simulink library "see_saw"  (R2013b)
settings: Solver=ode45  StartTime=0.0  StopTime=10.0  RelTol=1e-3
undefined symbols (not defined in the file): DiscIntNeverNeededParam, gcbh, K, R, realtime
libraries: legonxtlib x9
(part 1 of 2)
settings Model: Creator=mbiesiad  LastModifiedBy=grouleau

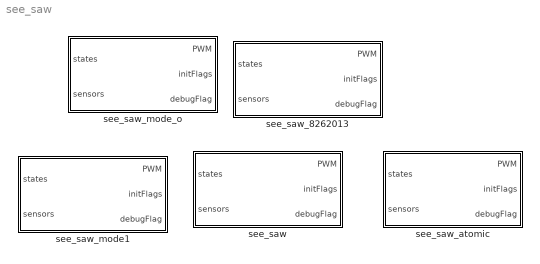
== system see_saw ==
  see_saw : Stateflow chart  TreatAsAtomicUnit=on
  see_saw_8262013 : Stateflow chart  TreatAsAtomicUnit=on
  see_saw_atomic : Stateflow chart  TreatAsAtomicUnit=on
  see_saw_mode1 : Stateflow chart  TreatAsAtomicUnit=on
  see_saw_mode_o : Stateflow chart  TreatAsAtomicUnit=on

== system see_saw/see_saw/see_saw_mode.DispTheta ==
  light : Inport  OutDataTypeStr=double  PortDimensions=1
  turningPWM : Inport  Port=2  OutDataTypeStr=double  PortDimensions=1
  f : TriggerPort  TriggerType=function-call
      settings: CopyFcn=Stateflow.SLINSF.SimulinkMan.removeBlockPreDeleteFcn  PreDeleteFcn=Stateflow.SLINSF.SimulinkMan.unsafePredeleteFcn
  Gain : Gain  Gain=100
  Gain1 : Gain  Gain=100
  LCD : legonxtlib/LCD  slcdStr=Theta  slcdLine=2  slcdFormat=Decimal
  LCD1 : Subsystem  InitFcn=realtime.validateBlock('LEGO MINDSTORMS NXT', gcbh, '')  mask(LEGO MINDSTORMS NXT LCD){slcdStr=turnPWM, slcdLine=3, slcdFormat=Decimal}
      mask prompts: slcdStr "Display label (maximum  8 characters):"; slcdLine "Display at line:"; slcdFormat "Display format:"
      mask help: Displays the numeric value from the block input port. The display truncates the input value to show only the integer portion. Use Display at line parameter to select the row. Use Display format parameter to select the format of the number: decimal or hexadecimal.
      mask init:
      | realtime.internal.nxtLcdSysCallback;
      mask Help: eval('realtime.helpView(''LEGO MINDSTORMS NXT'', ''legonxtlibnxtlcd'')')
      mask TypeOptions slcdLine: 1 | 2 | 3 | 4 | 5 | 6 | 7 | 8
      mask TypeOptions slcdFormat: Decimal | Hex
      mask Display:
      | [data, map]=imread('LCD.gif');pic=ind2rgb(data,map);image(pic,[0.32 0.25 0.35 0.55]);
      | lineText = sprintf('Line %d', slcdLine);
      | text(0.5, 0.15, lineText, 'horizontalAlignment', 'center');
      | port_label('input', 1, '');
      | color('blue');
      | text(0.65, 0.87, 'LEGO', 'horizontalAlignment', 'left');
  wires:
  Gain/1 -> LCD/1
  light/1 -> Gain/1
  Gain1/1 -> LCD1/1(In1)
  turningPWM/1 -> Gain1/1

== system see_saw/see_saw/see_saw_mode.Speak ==
  f : TriggerPort  TriggerType=function-call
      settings: CopyFcn=Stateflow.SLINSF.SimulinkMan.removeBlockPreDeleteFcn  PreDeleteFcn=Stateflow.SLINSF.SimulinkMan.unsafePredeleteFcn
  Constant : Constant  Value=50
  Speaker : legonxtlib/Speaker  sinputMode=Volume only  sspeakerFreq=800  sspeakerVolume=50  sspeakerDuration=100
  wires:
  Constant/1 -> Speaker/1

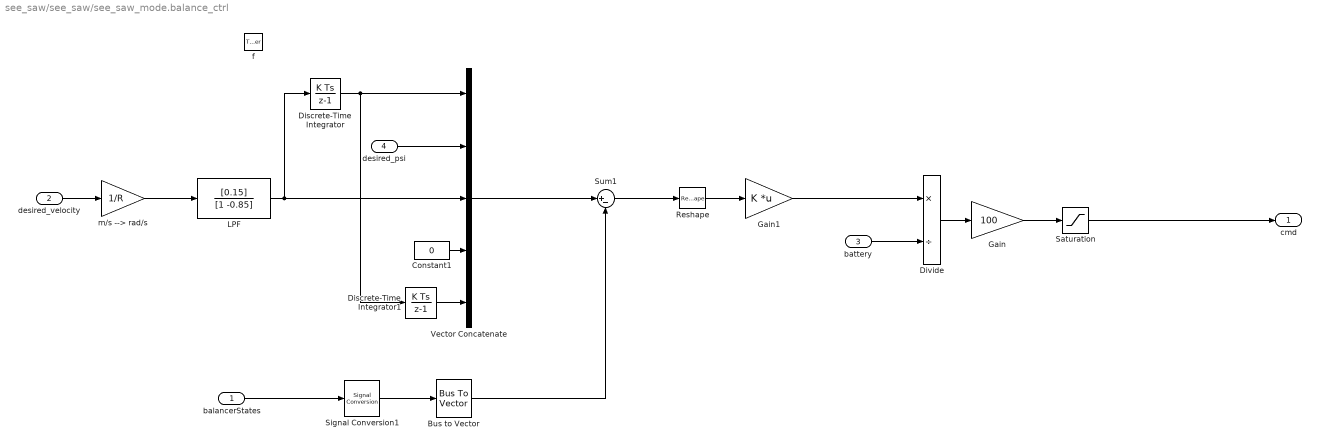
== system see_saw/see_saw/see_saw_mode.balance_ctrl ==
  balancerStates : Inport  OutDataTypeStr=Bus: Balancer_States_Bus  PortDimensions=1
  desired_velocity : Inport  Port=2  OutDataTypeStr=single  PortDimensions=1  BusOutputAsStruct=on
  battery : Inport  Port=3  OutDataTypeStr=double  PortDimensions=1
  desired_psi : Inport  Port=4  OutDataTypeStr=single  PortDimensions=1  BusOutputAsStruct=on
  f : TriggerPort  TriggerType=function-call
      settings: CopyFcn=Stateflow.SLINSF.SimulinkMan.removeBlockPreDeleteFcn  PreDeleteFcn=Stateflow.SLINSF.SimulinkMan.unsafePredeleteFcn
  Bus to Vector : BusToVector
  Constant1 : Constant  Value=0  OutDataTypeStr=single
  Discrete-Time Integrator : DiscreteIntegrator  SampleTime=-1  ICPrevOutput=DiscIntNeverNeededParam  ICPrevScaledInput=DiscIntNeverNeededParam
  Discrete-Time Integrator1 : DiscreteIntegrator  SampleTime=-1  ICPrevOutput=DiscIntNeverNeededParam  ICPrevScaledInput=DiscIntNeverNeededParam
  Divide : Product  Inputs=*/
  Gain : Gain  Gain=100
  Gain1 : Gain  Gain=K  Multiplication=Matrix(K*u)
  LPF : DiscreteFilter  Numerator=[0.15]  Denominator=[1 -0.85]
  Reshape : Reshape  OutputDimensionality=Column vector (2-D)
  Saturation : Saturate  UpperLimit=100  LowerLimit=-100  OutDataTypeStr=single
  Signal Conversion1 : SignalConversion  ConversionOutput=Virtual bus
  Sum1 : Sum  Inputs=|+-
  Vector Concatenate : Concatenate  NumInputs=5
  m/s --> rad/s : Gain  Gain=1/R
  cmd : Outport  OutDataTypeStr=single  PortDimensions=1  InitialOutput=0
  wires:
  Reshape/1 -> Gain1/1
  Sum1/1 -> Reshape/1
  desired_velocity/1 -> m/s --> rad/s/1
  Bus to Vector/1 -> Sum1/2
  balancerStates/1 -> Signal Conversion1/1
  Vector Concatenate/1 -> Sum1/1
  battery/1 -> Divide/2
  Saturation/1 -> cmd/1
  Gain1/1 -> Divide/1
  Gain/1 -> Saturation/1
  Divide/1 -> Gain/1
  Signal Conversion1/1 -> Bus to Vector/1
  m/s --> rad/s/1 -> LPF/1
  desired_psi/1 -> Vector Concatenate/2
  LPF/1 -> Discrete-Time Integrator/1, Vector Concatenate/3
  Constant1/1 -> Vector Concatenate/4
  Discrete-Time Integrator/1 -> Discrete-Time Integrator1/1, Vector Concatenate/1
  Discrete-Time Integrator1/1 -> Vector Concatenate/5

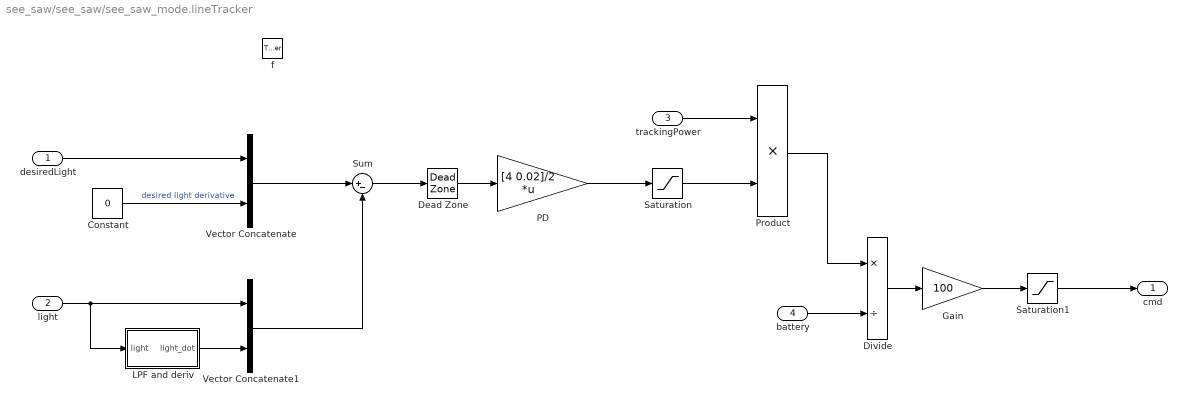
== system see_saw/see_saw/see_saw_mode.lineTracker ==
  desiredLight : Inport  OutDataTypeStr=single  PortDimensions=1
  light : Inport  Port=2  OutDataTypeStr=single  PortDimensions=1
  trackingPower : Inport  Port=3  OutDataTypeStr=single  PortDimensions=1
  battery : Inport  Port=4  OutDataTypeStr=double  PortDimensions=1
  f : TriggerPort  TriggerType=function-call
      settings: CopyFcn=Stateflow.SLINSF.SimulinkMan.removeBlockPreDeleteFcn  PreDeleteFcn=Stateflow.SLINSF.SimulinkMan.unsafePredeleteFcn
  Constant : Constant  Value=0  OutDataTypeStr=single
  Dead Zone : DeadZone  LowerValue=-0.02  UpperValue=0.02  SaturateOnIntegerOverflow=on
  Divide : Product  Inputs=*/
  Gain : Gain  Gain=100
  LPF and deriv : Subsystem
  PD : Gain  Gain="[4  0.02]/2"  Multiplication=Matrix(K*u)
  Product : Product
  Saturation : Saturate  UpperLimit=6  LowerLimit=-6
  Saturation1 : Saturate  UpperLimit=100  LowerLimit=-100  OutDataTypeStr=single
  Sum : Sum  Inputs=|+-
  Vector Concatenate : Concatenate
  Vector Concatenate1 : Concatenate
  cmd : Outport  OutDataTypeStr=single  PortDimensions=1
  wires:
  desiredLight/1 -> Vector Concatenate/1
  Constant/1 -> Vector Concatenate/2  "desired light derivative"
  LPF and deriv/1(light_dot) -> Vector Concatenate1/2
  light/1 -> LPF and deriv/1(light), Vector Concatenate1/1
  Vector Concatenate/1 -> Sum/1
  Vector Concatenate1/1 -> Sum/2
  Sum/1 -> Dead Zone/1
  Dead Zone/1 -> PD/1
  PD/1 -> Saturation/1
  Saturation/1 -> Product/2
  trackingPower/1 -> Product/1
  Product/1 -> Divide/1
  battery/1 -> Divide/2
  Gain/1 -> Saturation1/1
  Divide/1 -> Gain/1
  Saturation1/1 -> cmd/1

== system see_saw/see_saw/see_saw_mode.phiController ==
  phi : Inport  OutDataTypeStr=single  PortDimensions=1
  desiredPhi : Inport  Port=2  OutDataTypeStr=single  PortDimensions=1
  battery : Inport  Port=3  OutDataTypeStr=double  PortDimensions=1
  f : TriggerPort  TriggerType=function-call
      settings: CopyFcn=Stateflow.SLINSF.SimulinkMan.removeBlockPreDeleteFcn  PreDeleteFcn=Stateflow.SLINSF.SimulinkMan.unsafePredeleteFcn
  Divide : Product  Inputs=*/
  Gain : Gain  Gain=10
  Gain1 : Gain  Gain=100
  Saturation1 : Saturate  UpperLimit=100  LowerLimit=-100  OutDataTypeStr=single
  Sum : Sum  Inputs=|+-
  cmd : Outport
  wires:
  desiredPhi/1 -> Sum/1
  phi/1 -> Sum/2
  Sum/1 -> Gain/1
  battery/1 -> Divide/2
  Gain1/1 -> Saturation1/1
  Divide/1 -> Gain1/1
  Gain/1 -> Divide/1
  Saturation1/1 -> cmd/1

== system see_saw/see_saw/see_saw_mode.processLight ==
  rawLight : Inport  OutDataTypeStr=single  PortDimensions=1
  lightCalib : Inport  Port=2  OutDataTypeStr=Bus: Light_Bus  PortDimensions=1
  f : TriggerPort  TriggerType=function-call
      settings: CopyFcn=Stateflow.SLINSF.SimulinkMan.removeBlockPreDeleteFcn  PreDeleteFcn=Stateflow.SLINSF.SimulinkMan.unsafePredeleteFcn
  Bus Selector : BusSelector  OutputSignals=black,white
  Gain : Gain  Gain=0.3
  Gain1 : Gain  Gain=1/100
  Sum : Sum  Inputs=|+-
  Sum1 : Sum  Inputs=|++
  Sum2 : Sum  Inputs=|+-
  light : Outport
  wires:
  lightCalib/1 -> Bus Selector/1
  Bus Selector/1 -> Sum/1  "<black>"
  Bus Selector/2 -> Sum1/2, Sum/2  "<white>"
  Sum/1 -> Gain/1
  Gain/1 -> Sum1/1
  rawLight/1 -> Sum2/1
  Sum1/1 -> Sum2/2
  Sum2/1 -> Gain1/1
  Gain1/1 -> light/1

== system see_saw/see_saw/see_saw_mode.tail_controller ==
  note: Could be improved, PI for example
  current : Inport  OutDataTypeStr=single  PortDimensions=1
  desired : Inport  Port=2  OutDataTypeStr=single  PortDimensions=1
  f : TriggerPort  TriggerType=function-call
      settings: CopyFcn=Stateflow.SLINSF.SimulinkMan.removeBlockPreDeleteFcn  PreDeleteFcn=Stateflow.SLINSF.SimulinkMan.unsafePredeleteFcn
  Gain : Gain  Gain=250
  Saturation : Saturate  UpperLimit=100  LowerLimit=-100  OutDataTypeStr=single
  Sum : Sum  Inputs=|+-
  cmd : Outport  OutDataTypeStr=single  PortDimensions=1  InitialOutput=0
  wires:
  Sum/1 -> Gain/1
  current/1 -> Sum/2
  desired/1 -> Sum/1
  Gain/1 -> Saturation/1
  Saturation/1 -> cmd/1

== system see_saw/see_saw_8262013/see_saw_mode.DispTheta ==
  theta : Inport  OutDataTypeStr=double  PortDimensions=1
  f : TriggerPort  TriggerType=function-call
      settings: CopyFcn=Stateflow.SLINSF.SimulinkMan.removeBlockPreDeleteFcn  PreDeleteFcn=Stateflow.SLINSF.SimulinkMan.unsafePredeleteFcn
  Gain : Gain  Gain=100
  LCD : legonxtlib/LCD  slcdStr=Theta  slcdLine=2  slcdFormat=Decimal
  wires:
  theta/1 -> Gain/1
  Gain/1 -> LCD/1

== system see_saw/see_saw_8262013/see_saw_mode.Speak ==
  f : TriggerPort  TriggerType=function-call
      settings: CopyFcn=Stateflow.SLINSF.SimulinkMan.removeBlockPreDeleteFcn  PreDeleteFcn=Stateflow.SLINSF.SimulinkMan.unsafePredeleteFcn
  Constant : Constant  Value=50
  Speaker : legonxtlib/Speaker  sinputMode=Volume only  sspeakerFreq=800  sspeakerVolume=50  sspeakerDuration=100
  wires:
  Constant/1 -> Speaker/1

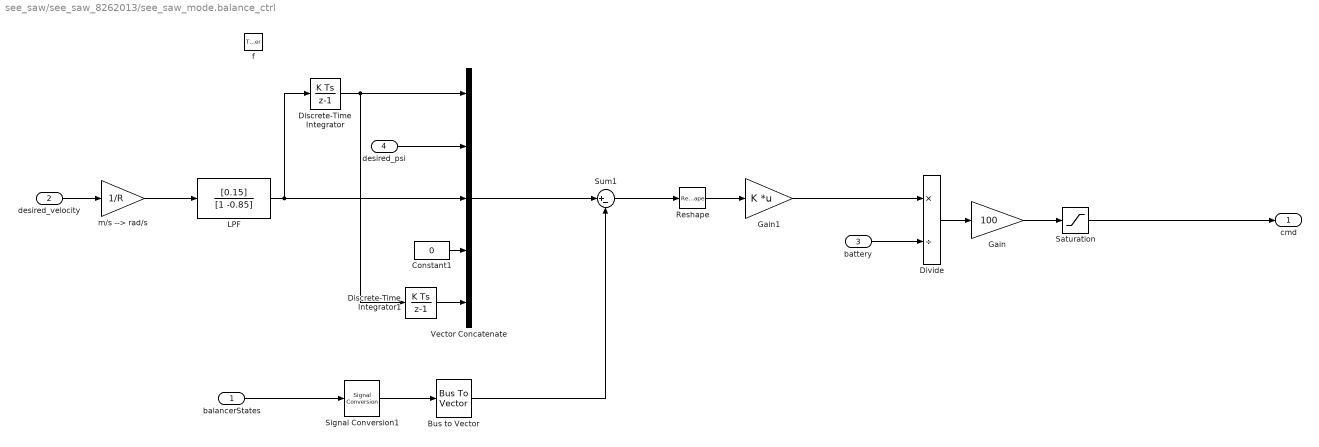
== system see_saw/see_saw_8262013/see_saw_mode.balance_ctrl ==
  balancerStates : Inport  OutDataTypeStr=Bus: Balancer_States_Bus  PortDimensions=1
  desired_velocity : Inport  Port=2  OutDataTypeStr=single  PortDimensions=1  BusOutputAsStruct=on
  battery : Inport  Port=3  OutDataTypeStr=double  PortDimensions=1
  desired_psi : Inport  Port=4  OutDataTypeStr=single  PortDimensions=1  BusOutputAsStruct=on
  f : TriggerPort  TriggerType=function-call
      settings: CopyFcn=Stateflow.SLINSF.SimulinkMan.removeBlockPreDeleteFcn  PreDeleteFcn=Stateflow.SLINSF.SimulinkMan.unsafePredeleteFcn
  Bus to Vector : BusToVector
  Constant1 : Constant  Value=0  OutDataTypeStr=single
  Discrete-Time Integrator : DiscreteIntegrator  SampleTime=-1  ICPrevOutput=DiscIntNeverNeededParam  ICPrevScaledInput=DiscIntNeverNeededParam
  Discrete-Time Integrator1 : DiscreteIntegrator  SampleTime=-1  ICPrevOutput=DiscIntNeverNeededParam  ICPrevScaledInput=DiscIntNeverNeededParam
  Divide : Product  Inputs=*/
  Gain : Gain  Gain=100
  Gain1 : Gain  Gain=K  Multiplication=Matrix(K*u)
  LPF : DiscreteFilter  Numerator=[0.15]  Denominator=[1 -0.85]
  Reshape : Reshape  OutputDimensionality=Column vector (2-D)
  Saturation : Saturate  UpperLimit=100  LowerLimit=-100  OutDataTypeStr=single
  Signal Conversion1 : SignalConversion  ConversionOutput=Virtual bus
  Sum1 : Sum  Inputs=|+-
  Vector Concatenate : Concatenate  NumInputs=5
  m/s --> rad/s : Gain  Gain=1/R
  cmd : Outport  OutDataTypeStr=single  PortDimensions=1  InitialOutput=0
  wires:
  Discrete-Time Integrator1/1 -> Vector Concatenate/5
  Discrete-Time Integrator/1 -> Vector Concatenate/1, Discrete-Time Integrator1/1
  Constant1/1 -> Vector Concatenate/4
  LPF/1 -> Vector Concatenate/3, Discrete-Time Integrator/1
  desired_psi/1 -> Vector Concatenate/2
  m/s --> rad/s/1 -> LPF/1
  Signal Conversion1/1 -> Bus to Vector/1
  Divide/1 -> Gain/1
  Gain/1 -> Saturation/1
  Gain1/1 -> Divide/1
  Saturation/1 -> cmd/1
  battery/1 -> Divide/2
  Vector Concatenate/1 -> Sum1/1
  balancerStates/1 -> Signal Conversion1/1
  Bus to Vector/1 -> Sum1/2
  desired_velocity/1 -> m/s --> rad/s/1
  Sum1/1 -> Reshape/1
  Reshape/1 -> Gain1/1

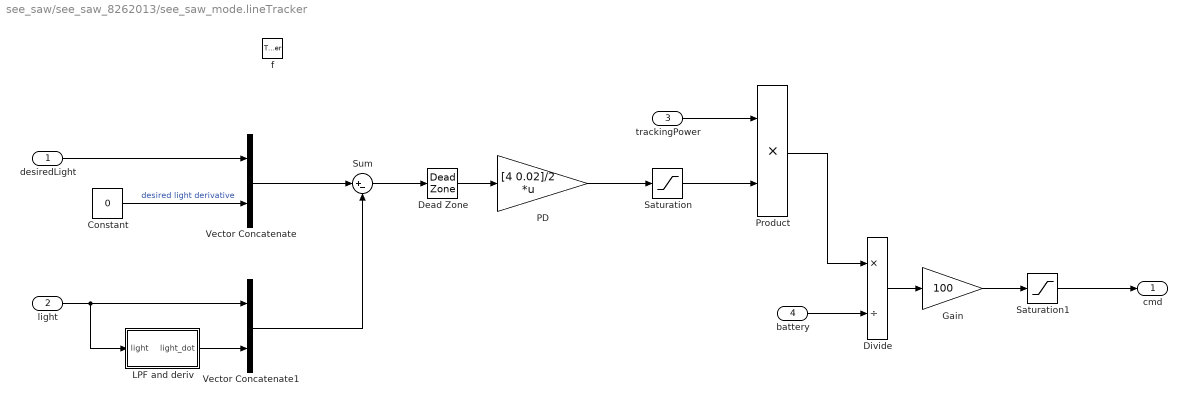
== system see_saw/see_saw_8262013/see_saw_mode.lineTracker ==
  desiredLight : Inport  OutDataTypeStr=single  PortDimensions=1
  light : Inport  Port=2  OutDataTypeStr=single  PortDimensions=1
  trackingPower : Inport  Port=3  OutDataTypeStr=single  PortDimensions=1
  battery : Inport  Port=4  OutDataTypeStr=double  PortDimensions=1
  f : TriggerPort  TriggerType=function-call
      settings: CopyFcn=Stateflow.SLINSF.SimulinkMan.removeBlockPreDeleteFcn  PreDeleteFcn=Stateflow.SLINSF.SimulinkMan.unsafePredeleteFcn
  Constant : Constant  Value=0  OutDataTypeStr=single
  Dead Zone : DeadZone  LowerValue=-0.02  UpperValue=0.02  SaturateOnIntegerOverflow=on
  Divide : Product  Inputs=*/
  Gain : Gain  Gain=100
  LPF and deriv : Subsystem
  PD : Gain  Gain="[4  0.02]/2"  Multiplication=Matrix(K*u)
  Product : Product
  Saturation : Saturate  UpperLimit=6  LowerLimit=-6
  Saturation1 : Saturate  UpperLimit=100  LowerLimit=-100  OutDataTypeStr=single
  Sum : Sum  Inputs=|+-
  Vector Concatenate : Concatenate
  Vector Concatenate1 : Concatenate
  cmd : Outport  OutDataTypeStr=single  PortDimensions=1
  wires:
  Saturation1/1 -> cmd/1
  Divide/1 -> Gain/1
  Gain/1 -> Saturation1/1
  battery/1 -> Divide/2
  Product/1 -> Divide/1
  trackingPower/1 -> Product/1
  Saturation/1 -> Product/2
  PD/1 -> Saturation/1
  Dead Zone/1 -> PD/1
  Sum/1 -> Dead Zone/1
  Vector Concatenate1/1 -> Sum/2
  Vector Concatenate/1 -> Sum/1
  light/1 -> Vector Concatenate1/1, LPF and deriv/1(light)
  LPF and deriv/1(light_dot) -> Vector Concatenate1/2
  Constant/1 -> Vector Concatenate/2  "desired light derivative"
  desiredLight/1 -> Vector Concatenate/1

== system see_saw/see_saw_8262013/see_saw_mode.phiController ==
  phi : Inport  OutDataTypeStr=single  PortDimensions=1
  desiredPhi : Inport  Port=2  OutDataTypeStr=single  PortDimensions=1
  battery : Inport  Port=3  OutDataTypeStr=double  PortDimensions=1
  f : TriggerPort  TriggerType=function-call
      settings: CopyFcn=Stateflow.SLINSF.SimulinkMan.removeBlockPreDeleteFcn  PreDeleteFcn=Stateflow.SLINSF.SimulinkMan.unsafePredeleteFcn
  Divide : Product  Inputs=*/
  Gain : Gain  Gain=10
  Gain1 : Gain  Gain=100
  Saturation1 : Saturate  UpperLimit=100  LowerLimit=-100  OutDataTypeStr=single
  Sum : Sum  Inputs=|+-
  cmd : Outport
  wires:
  Saturation1/1 -> cmd/1
  Gain/1 -> Divide/1
  Divide/1 -> Gain1/1
  Gain1/1 -> Saturation1/1
  battery/1 -> Divide/2
  Sum/1 -> Gain/1
  phi/1 -> Sum/2
  desiredPhi/1 -> Sum/1

== system see_saw/see_saw_8262013/see_saw_mode.processLight ==
  rawLight : Inport  OutDataTypeStr=single  PortDimensions=1
  lightCalib : Inport  Port=2  OutDataTypeStr=Bus: Light_Bus  PortDimensions=1
  f : TriggerPort  TriggerType=function-call
      settings: CopyFcn=Stateflow.SLINSF.SimulinkMan.removeBlockPreDeleteFcn  PreDeleteFcn=Stateflow.SLINSF.SimulinkMan.unsafePredeleteFcn
  Bus Selector : BusSelector  OutputSignals=black,white
  Gain : Gain  Gain=0.3
  Gain1 : Gain  Gain=1/100
  Sum : Sum  Inputs=|+-
  Sum1 : Sum  Inputs=|++
  Sum2 : Sum  Inputs=|+-
  light : Outport
  wires:
  Gain1/1 -> light/1
  Sum2/1 -> Gain1/1
  Sum1/1 -> Sum2/2
  rawLight/1 -> Sum2/1
  Gain/1 -> Sum1/1
  Sum/1 -> Gain/1
  Bus Selector/2 -> Sum/2, Sum1/2  "<white>"
  Bus Selector/1 -> Sum/1  "<black>"
  lightCalib/1 -> Bus Selector/1

== system see_saw/see_saw_8262013/see_saw_mode.tail_controller ==
  note: Could be improved, PI for example
  current : Inport  OutDataTypeStr=single  PortDimensions=1
  desired : Inport  Port=2  OutDataTypeStr=single  PortDimensions=1
  f : TriggerPort  TriggerType=function-call
      settings: CopyFcn=Stateflow.SLINSF.SimulinkMan.removeBlockPreDeleteFcn  PreDeleteFcn=Stateflow.SLINSF.SimulinkMan.unsafePredeleteFcn
  Gain : Gain  Gain=250
  Saturation : Saturate  UpperLimit=100  LowerLimit=-100  OutDataTypeStr=single
  Sum : Sum  Inputs=|+-
  cmd : Outport  OutDataTypeStr=single  PortDimensions=1  InitialOutput=0
  wires:
  Saturation/1 -> cmd/1
  Gain/1 -> Saturation/1
  desired/1 -> Sum/1
  current/1 -> Sum/2
  Sum/1 -> Gain/1

== system see_saw/see_saw_atomic/see_saw_mode.DispTheta ==
  light : Inport  OutDataTypeStr=double  PortDimensions=1
  turningPWM : Inport  Port=2  OutDataTypeStr=double  PortDimensions=1
  f : TriggerPort  TriggerType=function-call
      settings: CopyFcn=Stateflow.SLINSF.SimulinkMan.removeBlockPreDeleteFcn  PreDeleteFcn=Stateflow.SLINSF.SimulinkMan.unsafePredeleteFcn
  Gain : Gain  Gain=100
  Gain1 : Gain  Gain=100
  LCD : legonxtlib/LCD  slcdStr=Theta  slcdLine=2  slcdFormat=Decimal
  LCD1 : Subsystem  InitFcn=realtime.validateBlock('LEGO MINDSTORMS NXT', gcbh, '')  mask(LEGO MINDSTORMS NXT LCD){slcdStr=turnPWM, slcdLine=3, slcdFormat=Decimal}
      mask prompts: slcdStr "Display label (maximum  8 characters):"; slcdLine "Display at line:"; slcdFormat "Display format:"
      mask help: Displays the numeric value from the block input port. The display truncates the input value to show only the integer portion. Use Display at line parameter to select the row. Use Display format parameter to select the format of the number: decimal or hexadecimal.
      mask init:
      | realtime.internal.nxtLcdSysCallback;
      mask Help: eval('realtime.helpView(''LEGO MINDSTORMS NXT'', ''legonxtlibnxtlcd'')')
      mask TypeOptions slcdLine: 1 | 2 | 3 | 4 | 5 | 6 | 7 | 8
      mask TypeOptions slcdFormat: Decimal | Hex
      mask Display:
      | [data, map]=imread('LCD.gif');pic=ind2rgb(data,map);image(pic,[0.32 0.25 0.35 0.55]);
      | lineText = sprintf('Line %d', slcdLine);
      | text(0.5, 0.15, lineText, 'horizontalAlignment', 'center');
      | port_label('input', 1, '');
      | color('blue');
      | text(0.65, 0.87, 'LEGO', 'horizontalAlignment', 'left');
  wires:
  Gain/1 -> LCD/1
  light/1 -> Gain/1
  Gain1/1 -> LCD1/1(In1)
  turningPWM/1 -> Gain1/1

== system see_saw/see_saw_atomic/see_saw_mode.Speak ==
  f : TriggerPort  TriggerType=function-call
      settings: CopyFcn=Stateflow.SLINSF.SimulinkMan.removeBlockPreDeleteFcn  PreDeleteFcn=Stateflow.SLINSF.SimulinkMan.unsafePredeleteFcn
  Constant : Constant  Value=50
  Speaker : legonxtlib/Speaker  sinputMode=Volume only  sspeakerFreq=800  sspeakerVolume=50  sspeakerDuration=100
  wires:
  Constant/1 -> Speaker/1

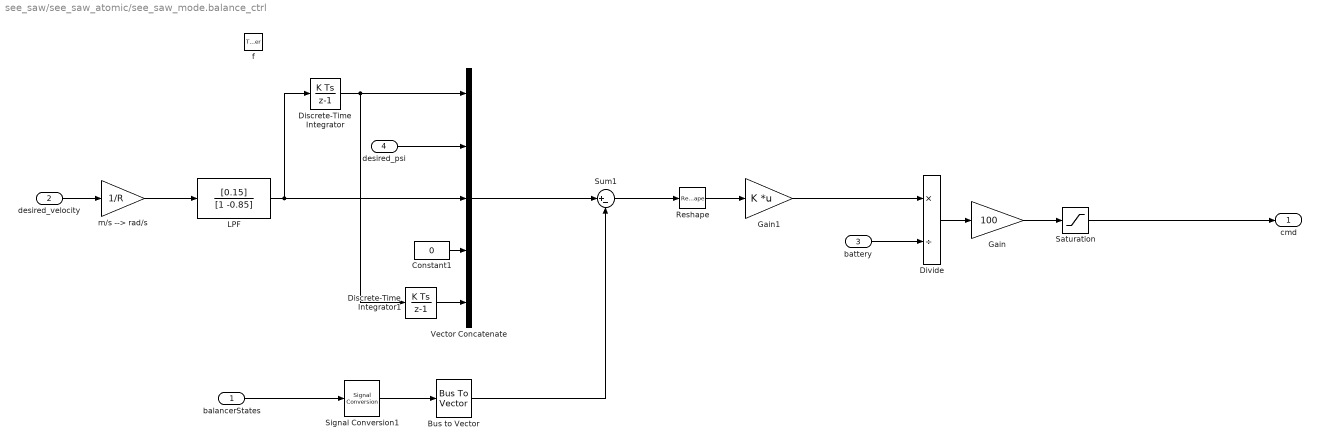
== system see_saw/see_saw_atomic/see_saw_mode.balance_ctrl ==
  balancerStates : Inport  OutDataTypeStr=Bus: Balancer_States_Bus  PortDimensions=1
  desired_velocity : Inport  Port=2  OutDataTypeStr=single  PortDimensions=1  BusOutputAsStruct=on
  battery : Inport  Port=3  OutDataTypeStr=double  PortDimensions=1
  desired_psi : Inport  Port=4  OutDataTypeStr=single  PortDimensions=1  BusOutputAsStruct=on
  f : TriggerPort  TriggerType=function-call
      settings: CopyFcn=Stateflow.SLINSF.SimulinkMan.removeBlockPreDeleteFcn  PreDeleteFcn=Stateflow.SLINSF.SimulinkMan.unsafePredeleteFcn
  Bus to Vector : BusToVector
  Constant1 : Constant  Value=0  OutDataTypeStr=single
  Discrete-Time Integrator : DiscreteIntegrator  SampleTime=-1  ICPrevOutput=DiscIntNeverNeededParam  ICPrevScaledInput=DiscIntNeverNeededParam
  Discrete-Time Integrator1 : DiscreteIntegrator  SampleTime=-1  ICPrevOutput=DiscIntNeverNeededParam  ICPrevScaledInput=DiscIntNeverNeededParam
  Divide : Product  Inputs=*/
  Gain : Gain  Gain=100
  Gain1 : Gain  Gain=K  Multiplication=Matrix(K*u)
  LPF : DiscreteFilter  Numerator=[0.15]  Denominator=[1 -0.85]
  Reshape : Reshape  OutputDimensionality=Column vector (2-D)
  Saturation : Saturate  UpperLimit=100  LowerLimit=-100  OutDataTypeStr=single
  Signal Conversion1 : SignalConversion  ConversionOutput=Virtual bus
  Sum1 : Sum  Inputs=|+-
  Vector Concatenate : Concatenate  NumInputs=5
  m/s --> rad/s : Gain  Gain=1/R
  cmd : Outport  OutDataTypeStr=single  PortDimensions=1  InitialOutput=0
  wires:
  Reshape/1 -> Gain1/1
  Sum1/1 -> Reshape/1
  desired_velocity/1 -> m/s --> rad/s/1
  Bus to Vector/1 -> Sum1/2
  balancerStates/1 -> Signal Conversion1/1
  Vector Concatenate/1 -> Sum1/1
  battery/1 -> Divide/2
  Saturation/1 -> cmd/1
  Gain1/1 -> Divide/1
  Gain/1 -> Saturation/1
  Divide/1 -> Gain/1
  Signal Conversion1/1 -> Bus to Vector/1
  m/s --> rad/s/1 -> LPF/1
  desired_psi/1 -> Vector Concatenate/2
  LPF/1 -> Discrete-Time Integrator/1, Vector Concatenate/3
  Constant1/1 -> Vector Concatenate/4
  Discrete-Time Integrator/1 -> Discrete-Time Integrator1/1, Vector Concatenate/1
  Discrete-Time Integrator1/1 -> Vector Concatenate/5

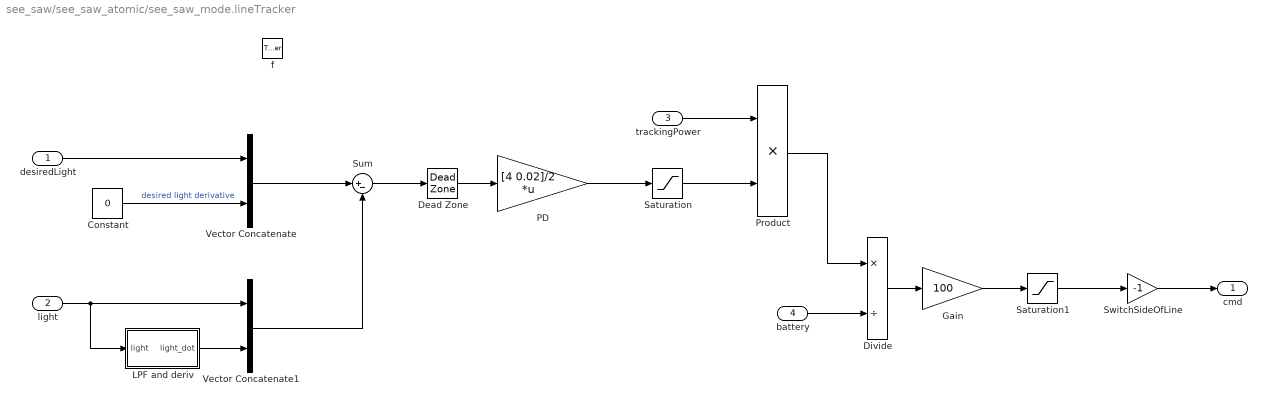
== system see_saw/see_saw_atomic/see_saw_mode.lineTracker ==
  desiredLight : Inport  OutDataTypeStr=single  PortDimensions=1
  light : Inport  Port=2  OutDataTypeStr=single  PortDimensions=1
  trackingPower : Inport  Port=3  OutDataTypeStr=single  PortDimensions=1
  battery : Inport  Port=4  OutDataTypeStr=double  PortDimensions=1
  f : TriggerPort  TriggerType=function-call
      settings: CopyFcn=Stateflow.SLINSF.SimulinkMan.removeBlockPreDeleteFcn  PreDeleteFcn=Stateflow.SLINSF.SimulinkMan.unsafePredeleteFcn
  Constant : Constant  Value=0  OutDataTypeStr=single
  Dead Zone : DeadZone  LowerValue=-0.02  UpperValue=0.02  SaturateOnIntegerOverflow=on
  Divide : Product  Inputs=*/
  Gain : Gain  Gain=100
  LPF and deriv : Subsystem
  PD : Gain  Gain="[4  0.02]/2"  Multiplication=Matrix(K*u)
  Product : Product
  Saturation : Saturate  UpperLimit=6  LowerLimit=-6
  Saturation1 : Saturate  UpperLimit=100  LowerLimit=-100  OutDataTypeStr=single
  Sum : Sum  Inputs=|+-
  SwitchSideOfLine : Gain  Gain=-1
  Vector Concatenate : Concatenate
  Vector Concatenate1 : Concatenate
  cmd : Outport  OutDataTypeStr=single  PortDimensions=1
  wires:
  SwitchSideOfLine/1 -> cmd/1
  desiredLight/1 -> Vector Concatenate/1
  Constant/1 -> Vector Concatenate/2  "desired light derivative"
  LPF and deriv/1(light_dot) -> Vector Concatenate1/2
  light/1 -> LPF and deriv/1(light), Vector Concatenate1/1
  Vector Concatenate/1 -> Sum/1
  Vector Concatenate1/1 -> Sum/2
  Sum/1 -> Dead Zone/1
  Dead Zone/1 -> PD/1
  PD/1 -> Saturation/1
  Saturation/1 -> Product/2
  trackingPower/1 -> Product/1
  Product/1 -> Divide/1
  battery/1 -> Divide/2
  Gain/1 -> Saturation1/1
  Divide/1 -> Gain/1
  Saturation1/1 -> SwitchSideOfLine/1

== system see_saw/see_saw_atomic/see_saw_mode.phiController ==
  phi : Inport  OutDataTypeStr=single  PortDimensions=1
  desiredPhi : Inport  Port=2  OutDataTypeStr=single  PortDimensions=1
  battery : Inport  Port=3  OutDataTypeStr=double  PortDimensions=1
  f : TriggerPort  TriggerType=function-call
      settings: CopyFcn=Stateflow.SLINSF.SimulinkMan.removeBlockPreDeleteFcn  PreDeleteFcn=Stateflow.SLINSF.SimulinkMan.unsafePredeleteFcn
  Divide : Product  Inputs=*/
  Gain : Gain  Gain=10
  Gain1 : Gain  Gain=100
  Saturation1 : Saturate  UpperLimit=100  LowerLimit=-100  OutDataTypeStr=single
  Sum : Sum  Inputs=|+-
  cmd : Outport
  wires:
  desiredPhi/1 -> Sum/1
  phi/1 -> Sum/2
  Sum/1 -> Gain/1
  battery/1 -> Divide/2
  Gain1/1 -> Saturation1/1
  Divide/1 -> Gain1/1
  Gain/1 -> Divide/1
  Saturation1/1 -> cmd/1

== system see_saw/see_saw_atomic/see_saw_mode.processLight ==
  rawLight : Inport  OutDataTypeStr=single  PortDimensions=1
  lightCalib : Inport  Port=2  OutDataTypeStr=Bus: Light_Bus  PortDimensions=1
  f : TriggerPort  TriggerType=function-call
      settings: CopyFcn=Stateflow.SLINSF.SimulinkMan.removeBlockPreDeleteFcn  PreDeleteFcn=Stateflow.SLINSF.SimulinkMan.unsafePredeleteFcn
  Bus Selector : BusSelector  OutputSignals=black,white
  Gain : Gain  Gain=0.3
  Gain1 : Gain  Gain=1/100
  Sum : Sum  Inputs=|+-
  Sum1 : Sum  Inputs=|++
  Sum2 : Sum  Inputs=|+-
  light : Outport
  wires:
  lightCalib/1 -> Bus Selector/1
  Bus Selector/1 -> Sum/1  "<black>"
  Bus Selector/2 -> Sum1/2, Sum/2  "<white>"
  Sum/1 -> Gain/1
  Gain/1 -> Sum1/1
  rawLight/1 -> Sum2/1
  Sum1/1 -> Sum2/2
  Sum2/1 -> Gain1/1
  Gain1/1 -> light/1

== system see_saw/see_saw_atomic/see_saw_mode.tail_controller ==
  note: Could be improved, PI for example
  current : Inport  OutDataTypeStr=single  PortDimensions=1
  desired : Inport  Port=2  OutDataTypeStr=single  PortDimensions=1
  f : TriggerPort  TriggerType=function-call
      settings: CopyFcn=Stateflow.SLINSF.SimulinkMan.removeBlockPreDeleteFcn  PreDeleteFcn=Stateflow.SLINSF.SimulinkMan.unsafePredeleteFcn
  Gain : Gain  Gain=250
  Saturation : Saturate  UpperLimit=100  LowerLimit=-100  OutDataTypeStr=single
  Sum : Sum  Inputs=|+-
  cmd : Outport  OutDataTypeStr=single  PortDimensions=1  InitialOutput=0
  wires:
  Sum/1 -> Gain/1
  current/1 -> Sum/2
  desired/1 -> Sum/1
  Gain/1 -> Saturation/1
  Saturation/1 -> cmd/1

== system see_saw/see_saw_mode1/see_saw_mode.Speak ==
  f : TriggerPort  TriggerType=function-call
      settings: CopyFcn=Stateflow.SLINSF.SimulinkMan.removeBlockPreDeleteFcn  PreDeleteFcn=Stateflow.SLINSF.SimulinkMan.unsafePredeleteFcn
  Constant : Constant  Value=50
  Speaker : legonxtlib/Speaker  sinputMode=Volume only  sspeakerFreq=800  sspeakerVolume=50  sspeakerDuration=100
  wires:
  Constant/1 -> Speaker/1

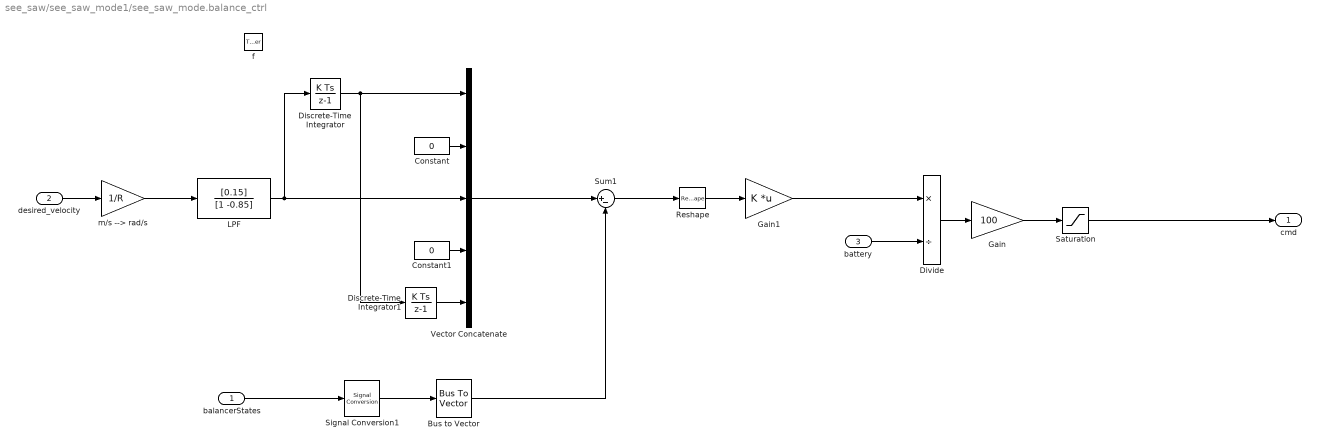
== system see_saw/see_saw_mode1/see_saw_mode.balance_ctrl ==
  balancerStates : Inport  OutDataTypeStr=Bus: Balancer_States_Bus  PortDimensions=1
  desired_velocity : Inport  Port=2  OutDataTypeStr=single  PortDimensions=1  BusOutputAsStruct=on
  battery : Inport  Port=3  OutDataTypeStr=double  PortDimensions=1
  f : TriggerPort  TriggerType=function-call
      settings: CopyFcn=Stateflow.SLINSF.SimulinkMan.removeBlockPreDeleteFcn  PreDeleteFcn=Stateflow.SLINSF.SimulinkMan.unsafePredeleteFcn
  Bus to Vector : BusToVector
  Constant : Constant  Value=0  OutDataTypeStr=single
  Constant1 : Constant  Value=0  OutDataTypeStr=single
  Discrete-Time Integrator : DiscreteIntegrator  SampleTime=-1  ICPrevOutput=DiscIntNeverNeededParam  ICPrevScaledInput=DiscIntNeverNeededParam
  Discrete-Time Integrator1 : DiscreteIntegrator  SampleTime=-1  ICPrevOutput=DiscIntNeverNeededParam  ICPrevScaledInput=DiscIntNeverNeededParam
  Divide : Product  Inputs=*/
  Gain : Gain  Gain=100
  Gain1 : Gain  Gain=K  Multiplication=Matrix(K*u)
  LPF : DiscreteFilter  Numerator=[0.15]  Denominator=[1 -0.85]
  Reshape : Reshape  OutputDimensionality=Column vector (2-D)
  Saturation : Saturate  UpperLimit=100  LowerLimit=-100  OutDataTypeStr=single
  Signal Conversion1 : SignalConversion  ConversionOutput=Virtual bus
  Sum1 : Sum  Inputs=|+-
  Vector Concatenate : Concatenate  NumInputs=5
  m/s --> rad/s : Gain  Gain=1/R
  cmd : Outport  OutDataTypeStr=single  PortDimensions=1  InitialOutput=0
  wires:
  Discrete-Time Integrator1/1 -> Vector Concatenate/5
  Discrete-Time Integrator/1 -> Vector Concatenate/1, Discrete-Time Integrator1/1
  Constant1/1 -> Vector Concatenate/4
  LPF/1 -> Vector Concatenate/3, Discrete-Time Integrator/1
  Constant/1 -> Vector Concatenate/2
  m/s --> rad/s/1 -> LPF/1
  Signal Conversion1/1 -> Bus to Vector/1
  Divide/1 -> Gain/1
  Gain/1 -> Saturation/1
  Gain1/1 -> Divide/1
  Saturation/1 -> cmd/1
  battery/1 -> Divide/2
  Vector Concatenate/1 -> Sum1/1
  balancerStates/1 -> Signal Conversion1/1
  Bus to Vector/1 -> Sum1/2
  desired_velocity/1 -> m/s --> rad/s/1
  Sum1/1 -> Reshape/1
  Reshape/1 -> Gain1/1

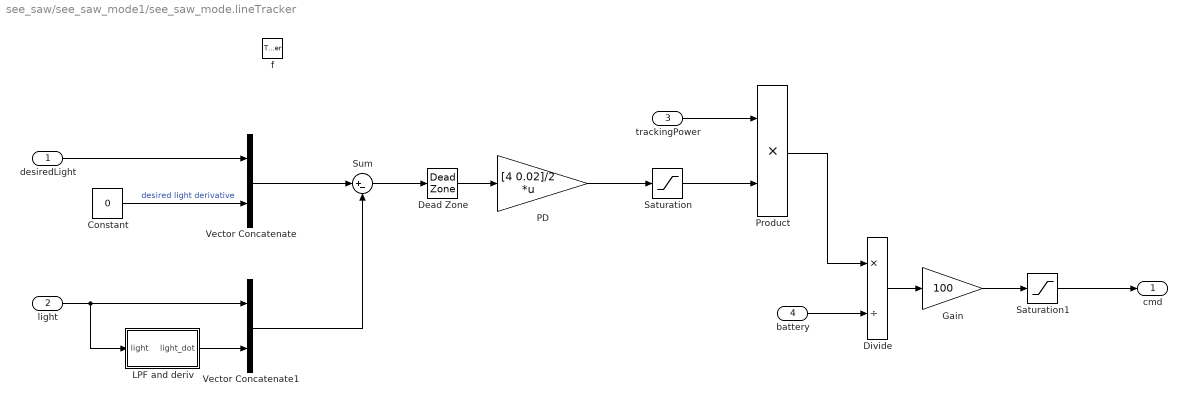
== system see_saw/see_saw_mode1/see_saw_mode.lineTracker ==
  desiredLight : Inport  OutDataTypeStr=single  PortDimensions=1
  light : Inport  Port=2  OutDataTypeStr=single  PortDimensions=1
  trackingPower : Inport  Port=3  OutDataTypeStr=single  PortDimensions=1
  battery : Inport  Port=4  OutDataTypeStr=double  PortDimensions=1
  f : TriggerPort  TriggerType=function-call
      settings: CopyFcn=Stateflow.SLINSF.SimulinkMan.removeBlockPreDeleteFcn  PreDeleteFcn=Stateflow.SLINSF.SimulinkMan.unsafePredeleteFcn
  Constant : Constant  Value=0  OutDataTypeStr=single
  Dead Zone : DeadZone  LowerValue=-0.02  UpperValue=0.02  SaturateOnIntegerOverflow=on
  Divide : Product  Inputs=*/
  Gain : Gain  Gain=100
  LPF and deriv : Subsystem
  PD : Gain  Gain="[4  0.02]/2"  Multiplication=Matrix(K*u)
  Product : Product
  Saturation : Saturate  UpperLimit=6  LowerLimit=-6
  Saturation1 : Saturate  UpperLimit=100  LowerLimit=-100  OutDataTypeStr=single
  Sum : Sum  Inputs=|+-
  Vector Concatenate : Concatenate
  Vector Concatenate1 : Concatenate
  cmd : Outport  OutDataTypeStr=single  PortDimensions=1
  wires:
  Saturation1/1 -> cmd/1
  Divide/1 -> Gain/1
  Gain/1 -> Saturation1/1
  battery/1 -> Divide/2
  Product/1 -> Divide/1
  trackingPower/1 -> Product/1
  Saturation/1 -> Product/2
  PD/1 -> Saturation/1
  Dead Zone/1 -> PD/1
  Sum/1 -> Dead Zone/1
  Vector Concatenate1/1 -> Sum/2
  Vector Concatenate/1 -> Sum/1
  light/1 -> Vector Concatenate1/1, LPF and deriv/1(light)
  LPF and deriv/1(light_dot) -> Vector Concatenate1/2
  Constant/1 -> Vector Concatenate/2  "desired light derivative"
  desiredLight/1 -> Vector Concatenate/1

== system see_saw/see_saw_mode1/see_saw_mode.phiController ==
  phi : Inport  OutDataTypeStr=single  PortDimensions=1
  desiredPhi : Inport  Port=2  OutDataTypeStr=single  PortDimensions=1
  battery : Inport  Port=3  OutDataTypeStr=double  PortDimensions=1
  f : TriggerPort  TriggerType=function-call
      settings: CopyFcn=Stateflow.SLINSF.SimulinkMan.removeBlockPreDeleteFcn  PreDeleteFcn=Stateflow.SLINSF.SimulinkMan.unsafePredeleteFcn
  Divide : Product  Inputs=*/
  Gain : Gain  Gain=10
  Gain1 : Gain  Gain=100
  Saturation1 : Saturate  UpperLimit=100  LowerLimit=-100  OutDataTypeStr=single
  Sum : Sum  Inputs=|+-
  cmd : Outport
  wires:
  Saturation1/1 -> cmd/1
  Gain/1 -> Divide/1
  Divide/1 -> Gain1/1
  Gain1/1 -> Saturation1/1
  battery/1 -> Divide/2
  Sum/1 -> Gain/1
  phi/1 -> Sum/2
  desiredPhi/1 -> Sum/1

== system see_saw/see_saw_mode1/see_saw_mode.processLight ==
  rawLight : Inport  OutDataTypeStr=single  PortDimensions=1
  lightCalib : Inport  Port=2  OutDataTypeStr=Bus: Light_Bus  PortDimensions=1
  f : TriggerPort  TriggerType=function-call
      settings: CopyFcn=Stateflow.SLINSF.SimulinkMan.removeBlockPreDeleteFcn  PreDeleteFcn=Stateflow.SLINSF.SimulinkMan.unsafePredeleteFcn
  Bus Selector : BusSelector  OutputSignals=black,white
  Gain : Gain  Gain=0.3
  Gain1 : Gain  Gain=1/100
  Sum : Sum  Inputs=|+-
  Sum1 : Sum  Inputs=|++
  Sum2 : Sum  Inputs=|+-
  light : Outport
  wires:
  Gain1/1 -> light/1
  Sum2/1 -> Gain1/1
  Sum1/1 -> Sum2/2
  rawLight/1 -> Sum2/1
  Gain/1 -> Sum1/1
  Sum/1 -> Gain/1
  Bus Selector/2 -> Sum/2, Sum1/2  "<white>"
  Bus Selector/1 -> Sum/1  "<black>"
  lightCalib/1 -> Bus Selector/1

== system see_saw/see_saw_mode1/see_saw_mode.tail_controller ==
  note: Could be improved, PI for example
  current : Inport  OutDataTypeStr=single  PortDimensions=1
  desired : Inport  Port=2  OutDataTypeStr=single  PortDimensions=1
  f : TriggerPort  TriggerType=function-call
      settings: CopyFcn=Stateflow.SLINSF.SimulinkMan.removeBlockPreDeleteFcn  PreDeleteFcn=Stateflow.SLINSF.SimulinkMan.unsafePredeleteFcn
  Gain : Gain  Gain=250
  Saturation : Saturate  UpperLimit=100  LowerLimit=-100  OutDataTypeStr=single
  Sum : Sum  Inputs=|+-
  cmd : Outport  OutDataTypeStr=single  PortDimensions=1  InitialOutput=0
  wires:
  Saturation/1 -> cmd/1
  Gain/1 -> Saturation/1
  desired/1 -> Sum/1
  current/1 -> Sum/2
  Sum/1 -> Gain/1

== system see_saw/see_saw_mode_o/see_saw_mode.DispTheta ==
  theta : Inport  OutDataTypeStr=double  PortDimensions=1
  f : TriggerPort  TriggerType=function-call
      settings: CopyFcn=Stateflow.SLINSF.SimulinkMan.removeBlockPreDeleteFcn  PreDeleteFcn=Stateflow.SLINSF.SimulinkMan.unsafePredeleteFcn
  Gain : Gain  Gain=100
  LCD : legonxtlib/LCD  slcdStr=Theta  slcdLine=2  slcdFormat=Decimal
  wires:
  Gain/1 -> LCD/1
  theta/1 -> Gain/1

== system see_saw/see_saw_mode_o/see_saw_mode.Speak ==
  f : TriggerPort  TriggerType=function-call
      settings: CopyFcn=Stateflow.SLINSF.SimulinkMan.removeBlockPreDeleteFcn  PreDeleteFcn=Stateflow.SLINSF.SimulinkMan.unsafePredeleteFcn
  Constant : Constant  Value=50
  Speaker : legonxtlib/Speaker  sinputMode=Volume only  sspeakerFreq=800  sspeakerVolume=50  sspeakerDuration=100
  wires:
  Constant/1 -> Speaker/1

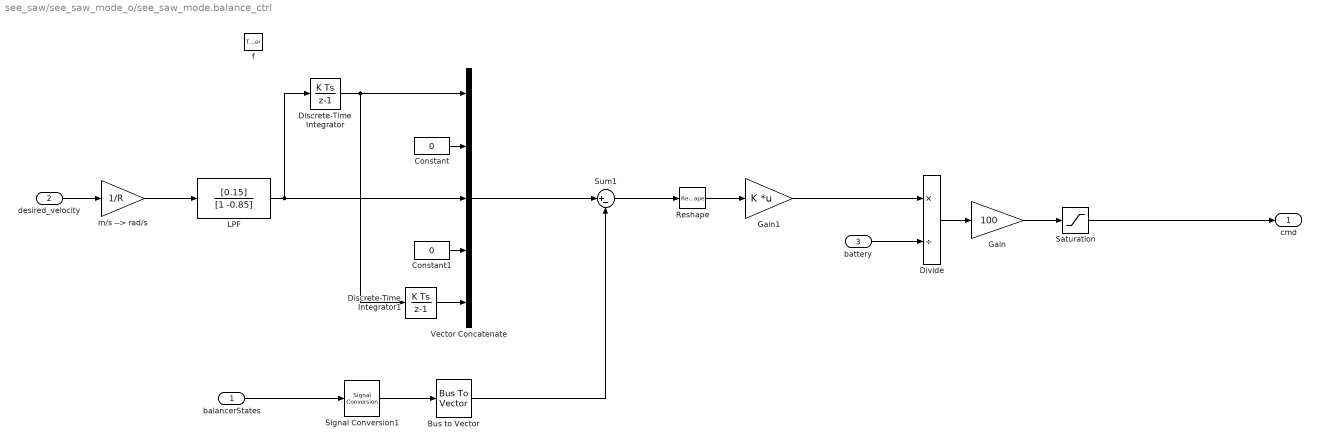
== system see_saw/see_saw_mode_o/see_saw_mode.balance_ctrl ==
  balancerStates : Inport  OutDataTypeStr=Bus: Balancer_States_Bus  PortDimensions=1
  desired_velocity : Inport  Port=2  OutDataTypeStr=single  PortDimensions=1  BusOutputAsStruct=on
  battery : Inport  Port=3  OutDataTypeStr=double  PortDimensions=1
  f : TriggerPort  TriggerType=function-call
      settings: CopyFcn=Stateflow.SLINSF.SimulinkMan.removeBlockPreDeleteFcn  PreDeleteFcn=Stateflow.SLINSF.SimulinkMan.unsafePredeleteFcn
  Bus to Vector : BusToVector
  Constant : Constant  Value=0  OutDataTypeStr=single
  Constant1 : Constant  Value=0  OutDataTypeStr=single
  Discrete-Time Integrator : DiscreteIntegrator  SampleTime=-1  ICPrevOutput=DiscIntNeverNeededParam  ICPrevScaledInput=DiscIntNeverNeededParam
  Discrete-Time Integrator1 : DiscreteIntegrator  SampleTime=-1  ICPrevOutput=DiscIntNeverNeededParam  ICPrevScaledInput=DiscIntNeverNeededParam
  Divide : Product  Inputs=*/
  Gain : Gain  Gain=100
  Gain1 : Gain  Gain=K  Multiplication=Matrix(K*u)
  LPF : DiscreteFilter  Numerator=[0.15]  Denominator=[1 -0.85]
  Reshape : Reshape  OutputDimensionality=Column vector (2-D)
  Saturation : Saturate  UpperLimit=100  LowerLimit=-100  OutDataTypeStr=single
  Signal Conversion1 : SignalConversion  ConversionOutput=Virtual bus
  Sum1 : Sum  Inputs=|+-
  Vector Concatenate : Concatenate  NumInputs=5
  m/s --> rad/s : Gain  Gain=1/R
  cmd : Outport  OutDataTypeStr=single  PortDimensions=1  InitialOutput=0
  wires:
  Reshape/1 -> Gain1/1
  Sum1/1 -> Reshape/1
  desired_velocity/1 -> m/s --> rad/s/1
  Bus to Vector/1 -> Sum1/2
  balancerStates/1 -> Signal Conversion1/1
  Vector Concatenate/1 -> Sum1/1
  battery/1 -> Divide/2
  Saturation/1 -> cmd/1
  Gain1/1 -> Divide/1
  Gain/1 -> Saturation/1
  Divide/1 -> Gain/1
  Signal Conversion1/1 -> Bus to Vector/1
  m/s --> rad/s/1 -> LPF/1
  Constant/1 -> Vector Concatenate/2
  LPF/1 -> Discrete-Time Integrator/1, Vector Concatenate/3
  Constant1/1 -> Vector Concatenate/4
  Discrete-Time Integrator/1 -> Discrete-Time Integrator1/1, Vector Concatenate/1
  Discrete-Time Integrator1/1 -> Vector Concatenate/5

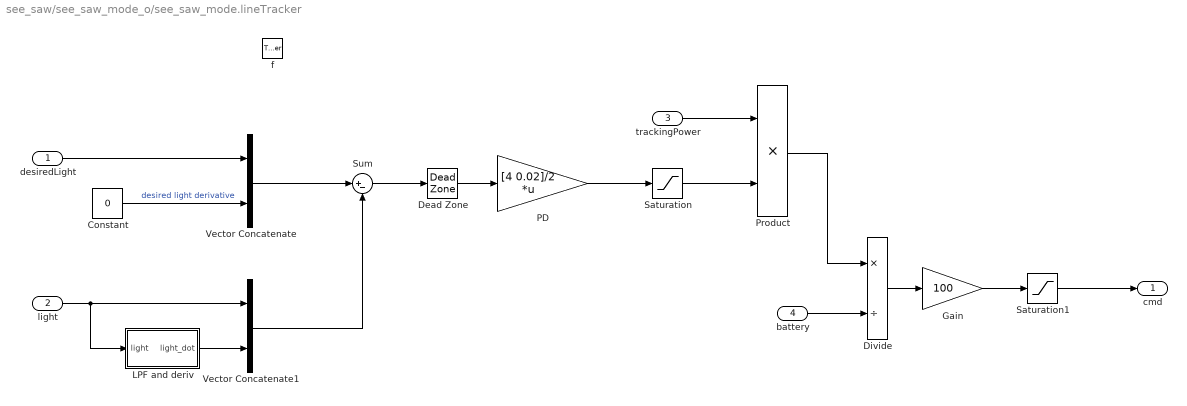
== system see_saw/see_saw_mode_o/see_saw_mode.lineTracker ==
  desiredLight : Inport  OutDataTypeStr=single  PortDimensions=1
  light : Inport  Port=2  OutDataTypeStr=single  PortDimensions=1
  trackingPower : Inport  Port=3  OutDataTypeStr=single  PortDimensions=1
  battery : Inport  Port=4  OutDataTypeStr=double  PortDimensions=1
  f : TriggerPort  TriggerType=function-call
      settings: CopyFcn=Stateflow.SLINSF.SimulinkMan.removeBlockPreDeleteFcn  PreDeleteFcn=Stateflow.SLINSF.SimulinkMan.unsafePredeleteFcn
  Constant : Constant  Value=0  OutDataTypeStr=single
  Dead Zone : DeadZone  LowerValue=-0.02  UpperValue=0.02  SaturateOnIntegerOverflow=on
  Divide : Product  Inputs=*/
  Gain : Gain  Gain=100
  LPF and deriv : Subsystem
  PD : Gain  Gain="[4  0.02]/2"  Multiplication=Matrix(K*u)
  Product : Product
  Saturation : Saturate  UpperLimit=6  LowerLimit=-6
  Saturation1 : Saturate  UpperLimit=100  LowerLimit=-100  OutDataTypeStr=single
  Sum : Sum  Inputs=|+-
  Vector Concatenate : Concatenate
  Vector Concatenate1 : Concatenate
  cmd : Outport  OutDataTypeStr=single  PortDimensions=1
  wires:
  desiredLight/1 -> Vector Concatenate/1
  Constant/1 -> Vector Concatenate/2  "desired light derivative"
  LPF and deriv/1(light_dot) -> Vector Concatenate1/2
  light/1 -> LPF and deriv/1(light), Vector Concatenate1/1
  Vector Concatenate/1 -> Sum/1
  Vector Concatenate1/1 -> Sum/2
  Sum/1 -> Dead Zone/1
  Dead Zone/1 -> PD/1
  PD/1 -> Saturation/1
  Saturation/1 -> Product/2
  trackingPower/1 -> Product/1
  Product/1 -> Divide/1
  battery/1 -> Divide/2
  Gain/1 -> Saturation1/1
  Divide/1 -> Gain/1
  Saturation1/1 -> cmd/1

== system see_saw/see_saw_mode_o/see_saw_mode.phiController ==
  phi : Inport  OutDataTypeStr=single  PortDimensions=1
  desiredPhi : Inport  Port=2  OutDataTypeStr=single  PortDimensions=1
  battery : Inport  Port=3  OutDataTypeStr=double  PortDimensions=1
  f : TriggerPort  TriggerType=function-call
      settings: CopyFcn=Stateflow.SLINSF.SimulinkMan.removeBlockPreDeleteFcn  PreDeleteFcn=Stateflow.SLINSF.SimulinkMan.unsafePredeleteFcn
  Divide : Product  Inputs=*/
  Gain : Gain  Gain=10
  Gain1 : Gain  Gain=100
  Saturation1 : Saturate  UpperLimit=100  LowerLimit=-100  OutDataTypeStr=single
  Sum : Sum  Inputs=|+-
  cmd : Outport
  wires:
  desiredPhi/1 -> Sum/1
  phi/1 -> Sum/2
  Sum/1 -> Gain/1
  battery/1 -> Divide/2
  Gain1/1 -> Saturation1/1
  Divide/1 -> Gain1/1
  Gain/1 -> Divide/1
  Saturation1/1 -> cmd/1

== system see_saw/see_saw_mode_o/see_saw_mode.processLight ==
  rawLight : Inport  OutDataTypeStr=single  PortDimensions=1
  lightCalib : Inport  Port=2  OutDataTypeStr=Bus: Light_Bus  PortDimensions=1
  f : TriggerPort  TriggerType=function-call
      settings: CopyFcn=Stateflow.SLINSF.SimulinkMan.removeBlockPreDeleteFcn  PreDeleteFcn=Stateflow.SLINSF.SimulinkMan.unsafePredeleteFcn
  Bus Selector : BusSelector  OutputSignals=black,white
  Gain : Gain  Gain=0.3
  Gain1 : Gain  Gain=1/100
  Sum : Sum  Inputs=|+-
  Sum1 : Sum  Inputs=|++
  Sum2 : Sum  Inputs=|+-
  light : Outport
  wires:
  lightCalib/1 -> Bus Selector/1
  Bus Selector/1 -> Sum/1  "<black>"
  Bus Selector/2 -> Sum1/2, Sum/2  "<white>"
  Sum/1 -> Gain/1
  Gain/1 -> Sum1/1
  rawLight/1 -> Sum2/1
  Sum1/1 -> Sum2/2
  Sum2/1 -> Gain1/1
  Gain1/1 -> light/1

== system see_saw/see_saw_mode_o/see_saw_mode.tail_controller ==
  note: Could be improved, PI for example
  current : Inport  OutDataTypeStr=single  PortDimensions=1
  desired : Inport  Port=2  OutDataTypeStr=single  PortDimensions=1
  f : TriggerPort  TriggerType=function-call
      settings: CopyFcn=Stateflow.SLINSF.SimulinkMan.removeBlockPreDeleteFcn  PreDeleteFcn=Stateflow.SLINSF.SimulinkMan.unsafePredeleteFcn
  Gain : Gain  Gain=250
  Saturation : Saturate  UpperLimit=100  LowerLimit=-100  OutDataTypeStr=single
  Sum : Sum  Inputs=|+-
  cmd : Outport  OutDataTypeStr=single  PortDimensions=1  InitialOutput=0
  wires:
  Sum/1 -> Gain/1
  current/1 -> Sum/2
  desired/1 -> Sum/1
  Gain/1 -> Saturation/1
  Saturation/1 -> cmd/1

== system see_saw/see_saw/see_saw_mode.DispTheta/LCD1 ==
  In1 : Inport
  Data Type Conversion : DataTypeConversion  OutDataTypeStr=int32
  LCD : S-Function  FunctionName=nxt_lcd  Parameters=lcdStr1, lcdLine, lcdFormat  EnableBusSupport=off  mask(NXT LCD){lcdStr=turnPWM, lcdLine=3, lcdFormat=Decimal}
      mask prompts: lcdStr "Prefix String (MAX 8 Characters):"; lcdLine "Display at Line:"; lcdFormat "Display Format:"
      mask help: Displays a number on NXT LCD screen
      mask init:
      | lcdStr1= [uint8(lcdStr) uint8(0)];
      mask TypeOptions lcdLine: 1 | 2 | 3 | 4 | 5 | 6 | 7 | 8
      mask TypeOptions lcdFormat: Decimal | Hex
      mask Display:
      | color('blue');
      | text(0.65, 0.87, 'LEGO', 'horizontalAlignment', 'left');
      | color('black');
      | port_label('input', 1, '');
  wires:
  Data Type Conversion/1 -> LCD/1
  In1/1 -> Data Type Conversion/1

== system see_saw/see_saw/see_saw_mode.lineTracker/LPF and deriv ==
  light : Inport
  Discrete Filter : DiscreteFilter  Numerator=[0.05]  Denominator=[1 -0.95]
  Gain : Gain  Gain=1/0.004
  Sum3 : Sum  Inputs=+-
  Unit Delay : UnitDelay  SampleTime=-1
  light_dot : Outport
  wires:
  light/1 -> Discrete Filter/1
  Discrete Filter/1 -> Gain/1
  Sum3/1 -> light_dot/1  "theta_dot_dot"
  Gain/1 -> Sum3/1, Unit Delay/1
  Unit Delay/1 -> Sum3/2

== system see_saw/see_saw_8262013/see_saw_mode.lineTracker/LPF and deriv ==
  light : Inport
  Discrete Filter : DiscreteFilter  Numerator=[0.05]  Denominator=[1 -0.95]
  Gain : Gain  Gain=1/0.004
  Sum3 : Sum  Inputs=+-
  Unit Delay : UnitDelay  SampleTime=-1
  light_dot : Outport
  wires:
  Unit Delay/1 -> Sum3/2
  Gain/1 -> Unit Delay/1, Sum3/1
  Sum3/1 -> light_dot/1  "theta_dot_dot"
  Discrete Filter/1 -> Gain/1
  light/1 -> Discrete Filter/1

== system see_saw/see_saw_atomic/see_saw_mode.DispTheta/LCD1 ==
  In1 : Inport
  Data Type Conversion : DataTypeConversion  OutDataTypeStr=int32
  LCD : S-Function  FunctionName=nxt_lcd  Parameters=lcdStr1, lcdLine, lcdFormat  EnableBusSupport=off  mask(NXT LCD){lcdStr=turnPWM, lcdLine=3, lcdFormat=Decimal}
      mask prompts: lcdStr "Prefix String (MAX 8 Characters):"; lcdLine "Display at Line:"; lcdFormat "Display Format:"
      mask help: Displays a number on NXT LCD screen
      mask init:
      | lcdStr1= [uint8(lcdStr) uint8(0)];
      mask TypeOptions lcdLine: 1 | 2 | 3 | 4 | 5 | 6 | 7 | 8
      mask TypeOptions lcdFormat: Decimal | Hex
      mask Display:
      | color('blue');
      | text(0.65, 0.87, 'LEGO', 'horizontalAlignment', 'left');
      | color('black');
      | port_label('input', 1, '');
  wires:
  Data Type Conversion/1 -> LCD/1
  In1/1 -> Data Type Conversion/1

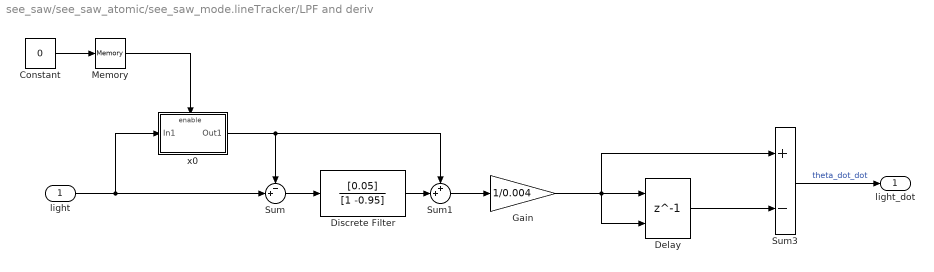
== system see_saw/see_saw_atomic/see_saw_mode.lineTracker/LPF and deriv ==
  light : Inport
  Constant : Constant  Value=0
  Delay : Delay  DelayLength=1  InitialConditionSource=Input port
      settings: InputPortMap=u0,p4
  Discrete Filter : DiscreteFilter  Numerator=[0.05]  Denominator=[1 -0.95]
  Gain : Gain  Gain=1/0.004
  Memory : Memory  X0=1  InheritSampleTime=on
  Sum : Sum  Inputs=-+|
  Sum1 : Sum  Inputs=++|
  Sum3 : Sum  Inputs=+-
  x0 : Subsystem  TreatAsAtomicUnit=on
  light_dot : Outport
  wires:
  Sum1/1 -> Gain/1
  Discrete Filter/1 -> Sum1/2
  x0/1(Out1) -> Sum/1, Sum1/1
  Sum/1 -> Discrete Filter/1
  Memory/1 -> x0/Enable
  Constant/1 -> Memory/1
  light/1 -> x0/1(In1), Sum/2
  Sum3/1 -> light_dot/1  "theta_dot_dot"
  Gain/1 -> Sum3/1, Delay/1, Delay/2
  Delay/1 -> Sum3/2

== system see_saw/see_saw_mode1/see_saw_mode.lineTracker/LPF and deriv ==
  light : Inport
  Discrete Filter : DiscreteFilter  Numerator=[0.05]  Denominator=[1 -0.95]
  Gain : Gain  Gain=1/0.004
  Sum3 : Sum  Inputs=+-
  Unit Delay : UnitDelay  SampleTime=-1
  light_dot : Outport
  wires:
  Unit Delay/1 -> Sum3/2
  Gain/1 -> Unit Delay/1, Sum3/1
  Sum3/1 -> light_dot/1  "theta_dot_dot"
  Discrete Filter/1 -> Gain/1
  light/1 -> Discrete Filter/1

== system see_saw/see_saw_mode_o/see_saw_mode.lineTracker/LPF and deriv ==
  light : Inport
  Discrete Filter : DiscreteFilter  Numerator=[0.05]  Denominator=[1 -0.95]
  Gain : Gain  Gain=1/0.004
  Sum3 : Sum  Inputs=+-
  Unit Delay : UnitDelay  SampleTime=-1
  light_dot : Outport
  wires:
  light/1 -> Discrete Filter/1
  Discrete Filter/1 -> Gain/1
  Sum3/1 -> light_dot/1  "theta_dot_dot"
  Gain/1 -> Sum3/1, Unit Delay/1
  Unit Delay/1 -> Sum3/2

== system see_saw/see_saw_atomic/see_saw_mode.lineTracker/LPF and deriv/x0 ==
  In1 : Inport
  Enable : EnablePort
  Out1 : Outport  InitialOutput=0
  wires:
  In1/1 -> Out1/1

== stateflow chart see_saw/see_saw_mode1 ==
  state see_saw_mode
    entry:
    desired_tail = single(1.6);
    during:
    normalizedLight = processLight(sensors.light,lightCalib);
    PWM.tail = tail_controller(sensors.theta_T, desired_tail);
    state light = processLight(rawLight,lightCalib) [function]
    state StandUp
      entry: debugFlag = uint16(602);
      initFlags.theta = single(1);
      initFlags.gyroReset = single(1);
      during:
      desired_tail = desired_tail + single(0.0008);
    state Balancing
      state SeesawLogic [parallel]
        settings: executionOrder=1
        state StationnaryBalance
          entry: debugFlag = uint16(603);
          desired_tail = single(0.5);
          initFlags.theta = single(0);
          initFlags.gyroReset = single(0);
          desired_states = balancerStates_Bus0;
        state Approach
          entry: debugFlag = uint16(604);
          during:
          turningPWM = lineTracker(single(-0.3), normalizedLight, single(1.3), sensors.battery);
          exit:
          turningPWM = single(0);
          state StartWalking
            entry:
            entry: debugFlag = uint16(605);
            des_vel = single(0.04);
            during:
            des_vel = des_vel+single(0.00024);
          state Walk
            entry: debugFlag = uint16(605);
          (default) -> StartWalking
          StartWalking -> Walk : [des_vel >= single(0.1)]
        state Seesaw
          state JumpOnIt
            entry:
            Speak;
            debugFlag = uint16(606);
            theta_ref = states.balancerStates.theta;
            phi_ref = states.phi;
            des_vel = single(0.15);
          state OnSeeSaw
            during:
            turningPWM = phiController(states.phi, phi_ref, sensors.battery);
            state GoingUP
              entry:
              entry: debugFlag = uint16(607);
              des_vel = single(0.1);
            state GoingBack
              entry:
              entry: debugFlag = uint16(607);
              des_vel = single(-0.1);
            state GoUpAgain
              entry:
              entry: debugFlag = uint16(607);
              des_vel = single(0.05);
            GoingUP -> GoingBack : [states.balancerStates.theta >= theta_ref + single(8.5)]
            GoingBack -> GoUpAgain : [states.balancerStates.theta <= theta_ref + single(6.5)]
          state Stop
            entry:
            entry: debugFlag = uint16(607);
            des_vel = single(0.05);
          (default) -> JumpOnIt
          JumpOnIt -> GoingUP : [states.balancerStates.theta >= theta_ref+single(1.57)]
          GoUpAgain -> Stop : [states.balancerStates.theta >= theta_ref + single(11.5)]
        state RaceDone
          entry: debugFlag = uint16(599);
          current_mode_status = OperationModeStatusEnum.SUCCESSFULLY_COMPLETED;
        (default) -> StationnaryBalance
        StationnaryBalance -> Approach : after(5,sec)
        Approach -> Seesaw : [states.balancerStates.theta_dot<single(-4)  && states.theta_dot_dot < single(-60) ]
      state After [parallel]
        during:
        forwardPWM = balance_ctrl(states.balancerStates, des_vel ,sensors.battery)
        PWM.left = forwardPWM - turningPWM;
        PWM.right = forwardPWM + turningPWM;
        settings: executionOrder=2
    state cmd = phiController(phi,desiredPhi,battery) [function]
    state cmd = lineTracker(desiredLight,light,trackingPower,battery) [function]
    state Speak [function]
    state cmd = tail_controller(current,desired) [function]
    state cmd = balance_ctrl(balancerStates,desired_velocity,battery) [function]
    (default) -> StandUp
    StandUp -> Balancing : [desired_tail >=single(2.0) && sensors.theta_T >= single(2.0)]
  data: rawLight function_input single size=1; lightCalib function_input Bus: Light_Bus size=1; light function_output; cmd function_output; phi function_input single size=1; desiredPhi function_input single size=1; battery function_input double size=1; cmd function_output single size=1; desiredLight function_input single size=1; light function_input single size=1; trackingPower function_input single size=1; battery function_input double size=1; current function_input single size=1; desired function_input single size=1; cmd function_output single size=1; balancerStates function_input Bus: Balancer_States_Bus size=1; desired_velocity function_input single size=1; battery function_input double size=1; cmd function_output single size=1; states input Bus: States_Bus size=1; sensors input Bus: Sensors_Bus size=1; PWM output Bus: PWM_bus size=1; initFlags output Bus: Init_Bus size=1; debugFlag output uint16 size=1; desired_states local Bus: Balancer_States_Bus size=1; desired_tail local single size=1; current_mode_status data_store_memory; balancerStates_Bus0 parameter Bus: Balancer_States_Bus size=1; lightCalib data_store_memory; normalizedLight local single size=1; des_vel local single size=1; theta_ref local single size=1; forwardPWM local single size=1; turningPWM local single size=1; phi_ref local single
